simulink model "System_v2"  (R2018b)
settings: Solver=VariableStepAuto  StartTime=0.0  StopTime=stopTime  MaxStep=maxStepSize  RelTol=1e-3
InitFcn:
  | InitialisationScript_v2
values from neighbouring files (symbols this model uses):
  a_turb = -7    [InitialisationScript.m]
  AlphaEvapSteam = 3500    [InitialisationScript.m]    (also in InitialisationScript_v2.m)
  AlphaSuperSteam = 70    [InitialisationScript.m]    (also in InitialisationScript_v2.m)
  CpumpEta = 0.75    [InitialisationScript.m]    (also in InitialisationScript_v2.m)
  eta_nom = 0.8    [InitialisationScript.m]
  evapFraction = 0.95    [InitialisationScript.m]    (also in InitialisationScript_v2.m = 0.938024869451)
  fuel_mass = 10000    [InitialisationScript.m]    (also in InitialisationScript_v2.m)
  h_max = 1000    [InitialisationScript_v2.m]
  k_pipe = 2e-3    (= 0.002)    [InitialisationScript_v2.m]
  N_min = 0.35    [InitialisationScript_v2.m]
  p1 = 18    [InitialisationScript.m]
  p2 = 0.6    [InitialisationScript.m]
  pipeLength = 4    [InitialisationScript.m]    (also in InitialisationScript_v2.m = 3.66)
  pressureFG = 50*9.81*1000    (= 490500)    [InitialisationScript_v2.m]
  Q_max = 52.254728179762466    (= 52.2547281798)    [InitialisationScript_v2.m]
  returnFGdelay = 3    [InitialisationScript.m]    (also in InitialisationScript_v2.m)
  rho_ethanole = 789    [InitialisationScript.m]    (also in InitialisationScript_v2.m)
  theta1_nom = 246.76    [InitialisationScript.m]
  theta_ret = 227.95    [InitialisationScript.m]    (also in InitialisationScript_v2.m)
  thetaFuelIn = 10    [InitialisationScript.m]    (also in InitialisationScript_v2.m)
  thetaO2In = 10    [InitialisationScript.m]    (also in InitialisationScript_v2.m)
undefined symbols (not defined in the file or in its folder): AinternalEvap, AinternalSuper, AwallEvap, AwallSuper, conductivity, extDiameter, K_stodola, qmd_ref, sub, thickness
libraries: simulink x1
settings Model: Creator=Danijel  LastModifiedBy=Danijel
settings DebuggingCC: UnderSpecifiedDimensionMsg=warning

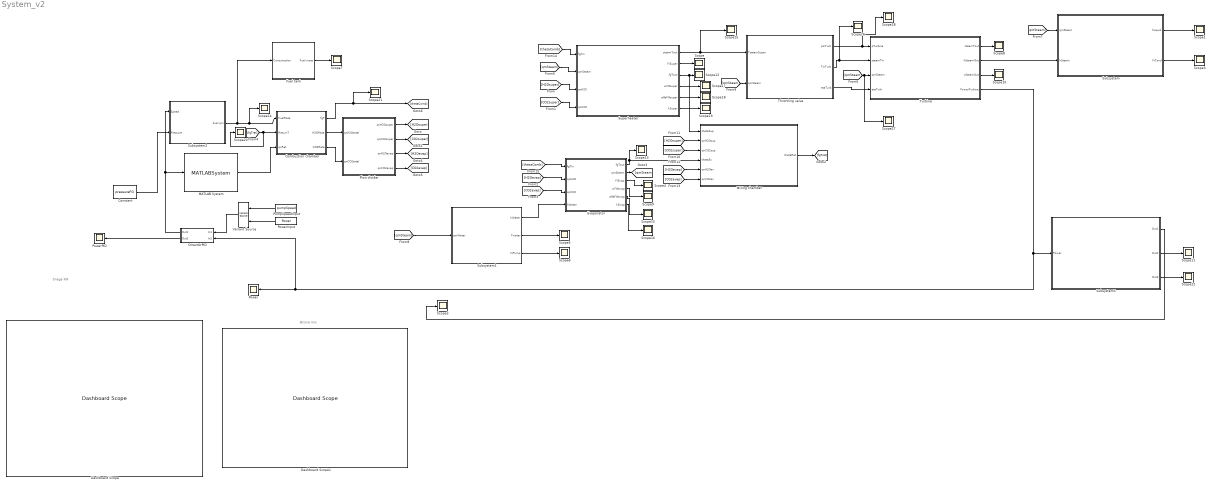
== system System_v2 ==
  note: Brzina m/s
  note: Snaga kW
  Combustion chamber : Subsystem  mask{thetaG_in=thetaFuelIn, thetaO2_in=thetaO2In, fgDelay=returnFGdelay, thetaRetInit=theta_ret}
      mask prompts: thetaG_in "Fuel temperature [°C]:"; thetaO2_in "Oxygen temperature [°C]:"; fgDelay "Flue gas return delay [s]"; thetaRetInit "Initial flue gas return temperature"
      mask help: Models fuel combustion with flue gas return
      mask TypeOptions thetaG_in: MATLAB System/thetaG_in
      mask TypeOptions thetaO2_in: MATLAB System/thetaO2_in
      mask DialogControl DescGroupVar Prompt: Combustion chamber
      mask Display: text(0.3,0.9, '{\bf\fontsize{12}Combustion}', 'texmode','on');
  Constant : Constant  Value=pressureFG
  DIrectOrPID : Subsystem  Variant=on
  Dashboard Scope : DashboardScope  Description=Turbine power  WebBlockId=277  Ymin=0  Ymax=110
  Dashboard Scope1 : DashboardScope  WebBlockId=358
  Evaporator : Subsystem  mask{p1=p1, A_evap=AwallEvap, flueGasFlowArea=AinternalEvap, pipeDiameterExternal=extDiameter, pipeThickness=thickness, AlfaS=AlphaEvapSteam, pipeConductivity=conductivity}
      mask prompts: p1 "Evaporation pressure [bar]:"; A_evap "Evaporator heat transfer area [m2]:"; flueGasFlowArea "Evaporator overall internal tube crossection area [m2]:"; pipeDiameterExternal "Evaporator pipe external diameter [m]:"; pipeThickness "Evaporator pipe thickness [m]:"; AlfaS "Evaporation heat transfer coefficient [W/m2K]:"; pipeConductivity "Tube material thermal conductivity [W/(mK)]:"
      mask help: Models steam evaporation. Calculates steam flow rate and flue gas outlet temperature.
      mask TypeOptions p1: MATLAB System2/p1
      mask TypeOptions A_evap: MATLAB System2/A_evap
      mask TypeOptions flueGasFlowArea: MATLAB System2/flueGasFlowArea
      mask TypeOptions pipeDiameterExternal: MATLAB System2/pipeDiameterExternal
      mask TypeOptions pipeThickness: MATLAB System2/pipeThickness
      mask TypeOptions AlfaS: MATLAB System2/AlfaS
      mask TypeOptions pipeConductivity: MATLAB System2/pipeConductivity
      mask DialogControl DescGroupVar Prompt: Evaporator
      mask Display: text(0.35,0.9, '{\bf\fontsize{12}Evaporator}', 'texmode','on');
  Flow divider : Subsystem  mask{evap_ratio=evapFraction}
      mask prompts: evap_ratio "Fraction of flue gases to evaporator [0-1]"
  Fuel tank : Subsystem  mask{InitialFuelMass=fuel_mass}
      mask prompts: InitialFuelMass "Initial fuel mass [kg]"
      mask Display: text(0.3,0.9, '{\bf\fontsize{12}Fuel tank}', 'texmode','on');
  MATLAB System : MATLABSystem  System=CompressorS  qmRetMin=qnRetMin  qmRetMax=qnRetMax  qmRetlow=qnRetlow  qmRethigh=qnRethigh  Nretlow=Nretlow  Nrethigh=Nrethigh  SimulateUsing=Code generation
      mask Type: CompressorS
      mask Display:
      | disp('CompressorS');
      | port_label('input',1,'N');
      | port_label('output',1,'qmRet');
  Mixing chamber : Subsystem
      mask Display: text(0.35,0.9, '{\bf\fontsize{12}Flue gas mix}', 'texmode','on');
  Power : Scope
  PowerInput : FromWorkspace  VariableName=Power  SampleTime=0
  PowerPID : Scope
  PumpSpeedInput : FromWorkspace  VariableName=pumpSpeed  SampleTime=0
  Scope{,1..22,25..28} (27 alike) : Scope
  Subsystem : Subsystem  mask{p2=p2}
      mask prompts: p2 "Condensation pressure [bar]:"
      mask help: Models steam condensation.
      mask TypeOptions p2: MATLAB System/p2
      mask DialogControl DescGroupVar Prompt: Condenser
      mask Display: text(0.4,0.9, '{\bf\fontsize{12}Condenser}', 'texmode','on');
  Subsystem1 : Subsystem  mask{p1=p1, p2=p2, eta=CpumpEta}
      mask prompts: p1 "Evaporation pressure [bar]:"; p2 "Condensation pressure [bar]:"; eta "Pump efficiency  [-]:"
      mask TypeOptions p1: MATLAB System/p1
      mask TypeOptions p2: MATLAB System/p2
      mask TypeOptions eta: MATLAB System/eta
      mask Display: text(0.27,0.92, '{\bf\fontsize{12}Condensate pump}', 'texmode','on');
  Subsystem2 : Subsystem  mask{Q_max=Q_max, h_max=h_max, n_min=N_min, rho_ethanole=rho_ethanole, k_pipe=k_pipe}
      mask prompts: Q_max "Fuel pump nominal volume flow rate [l/h]:"; h_max "Fuel pump nominal head [m]:"; n_min "Pump minimal relative speed [-]:"; rho_ethanole "Ethanole density [kg/m3]:"; k_pipe "pipe coefficient:"
      mask TypeOptions Q_max: MATLAB System/Q_max
      mask TypeOptions h_max: MATLAB System/h_max
      mask TypeOptions n_min: MATLAB System/n_min
      mask TypeOptions rho_ethanole: MATLAB System/rho_ethanole
      mask TypeOptions k_pipe: MATLAB System/k_pipe
      mask Display: text(0.3,0.9, '{\bf\fontsize{12}Fuel pump}', 'texmode','on');
  Subsystem3 : Subsystem
  Superheater : Subsystem  mask{p1=p1, A_super=AwallSuper, flueGasFlowArea=AinternalSuper, pipeDiameterExternal=extDiameter, pipeThickness=thickness, AlfaS=AlphaSuperSteam, pipeConductivity=conductivity, pipeLength=pipeLength}
      mask prompts: p1 "Evaporation pressure [bar]:"; A_super "Superheater heat transfer area [m2]:"; flueGasFlowArea "Superheater overall internal tube crossection area [m2]:"; pipeDiameterExternal "External pipe diameter [m]:"; pipeThickness "Superheater pipe thickness [m]:"; AlfaS "Superheating heat transfer coefficient [W/m2K]:"; pipeConductivity "Tube material thermal conductivity [W/(mK)]:"; pipeLength "Pipe length [m]:"
      mask help: Models steam superheating. Calculates outlet flue gas and steam temperatures.
      mask TypeOptions p1: MATLAB System3/p1
      mask TypeOptions A_super: MATLAB System3/A_super
      mask TypeOptions flueGasFlowArea: MATLAB System3/flueGasFlowArea
      mask TypeOptions pipeDiameterExternal: MATLAB System3/pipeDiameterExternal
      mask TypeOptions pipeThickness: MATLAB System3/pipeThickness
      mask TypeOptions AlfaS: MATLAB System3/AlfaS
      mask TypeOptions pipeConductivity: MATLAB System3/pipeConductivity
      mask TypeOptions pipeLength: MATLAB System3/pipeLength
      mask DialogControl DescGroupVar Prompt: Superheater
      mask Display: text(0.4,0.9, '{\bf\fontsize{12}Superheater}', 'texmode','on');
  Throttling valve : Subsystem  mask{p1=p1, p2=p2, theta1_nom=theta1_nom, qmd_nom=qmd_ref, eta_nom=eta_nom, a=a_turb, K=K_stodola}
      mask prompts: p1 "Evaporation pressure [bar]:"; p2 "Condensation pressure [bar]:"; theta1_nom "Nominal superheating temperature [°C]:"; qmd_nom "Nominal steam mass flow rate [kg/s]:"; eta_nom "Efficiency at nominal working conditions [-]:"; a "Quadratic efficiency coefficient:"; K "Stodola coefficient:"
      mask TypeOptions p1: MATLAB System/p1
      mask TypeOptions p2: MATLAB System/p2
      mask TypeOptions theta1_nom: MATLAB System/theta1_nom
      mask TypeOptions qmd_nom: MATLAB System/qmd_nom
      mask TypeOptions eta_nom: MATLAB System/eta_nom
      mask TypeOptions a: MATLAB System/a
      mask TypeOptions K: MATLAB System/K
      mask Display: text(0.35,0.9, '{\bf\fontsize{12}Throttling valve}', 'texmode','on');
  Turbine : Subsystem  mask{p_evap=p1, p2=p2}
      mask prompts: p_evap "Evaporation pressure [bar]:"; p2 "Condensation pressure [bar]:"
      mask help: Models steam expansion in tuebine. Calulates turbine power and outlet steam state.
      mask TypeOptions p_evap: MATLAB System4/p_evap
      mask TypeOptions p2: MATLAB System4/p2
      mask DialogControl DescGroupVar Prompt: Steam turbine
      mask Display: text(0.4,0.9, '{\bf\fontsize{12}Steam turbine}', 'texmode','on');
  Variant Source : VariantSource
  wires:
  [fgTret] -> Scope20/1, Combustion chamber/2(ReturnT)
  Evaporator/2(qmSteam) -> [qmSteam]
  [qmSteam] -> Superheater/2(qmSteam)
  Superheater/2(FiSuper) -> Scope/1
  [qmSteam] -> Scope27/1, Turbine/3(qmSteam)
  Turbine/1(steamTout) -> Scope8/1
  Turbine/3(xSteamOut) -> Scope10/1
  [qmSteam] -> Subsystem/1(qmSteam)
  Turbine/2(hSteamOut) -> Subsystem/2(hSteam)
  Subsystem/1(hLiquid) -> Scope1/1
  Subsystem/2(FiCond) -> Scope3/1
  Subsystem1/1(hWater) -> Evaporator/4(hWater)
  [qmSteam] -> Subsystem1/1(qmWater)
  Subsystem1/2(Twater) -> Scope5/1
  Subsystem1/3(FiPump) -> Scope6/1
  Fuel tank/1(Fuel mass) -> Scope7/1
  Superheater/1(steamTout) -> Scope25/1, Throttling valve/1(TsteamSuper)
  [qmSteam] -> Throttling valve/2(qmSteam)
  Throttling valve/1(pInTurb) -> Scope28/1, Turbine/1(pTurbine)
  Throttling valve/2(TinTurb) -> Scope26/1, Turbine/2(steamTin)
  Throttling valve/3(etaTurb) -> Turbine/4(etaTurb)
  Evaporator/1(fgTout) -> Mixing chamber/4(thetaEv), Scope13/1
  Superheater/3(fgTout) -> Mixing chamber/1(thetaSup), Scope12/1
  Combustion chamber/2(H2ORate) -> Flow divider/1(qnH2Ototal)
  Combustion chamber/3(CO2Rate) -> Flow divider/2(qnCO2total)
  Flow divider/1(qnH2Osuper) -> [H2Osuper]
  Flow divider/2(qnCO2super) -> [CO2super]
  Flow divider/3(qnH2Oevap) -> [H2Oevap]
  Flow divider/4(qnCO2evap) -> [CO2evap]
  [H2Osuper] -> Superheater/3(qnH20)
  [CO2super] -> Superheater/4(qnCO2)
  [H2Oevap] -> Evaporator/2(qnH2O)
  [CO2evap] -> Evaporator/3(qnCO2)
  [thetaComb] -> Superheater/1(fgTin)
  [thetaComb] -> Evaporator/1(fgTin)
  [H2Osuper] -> Mixing chamber/2(qnH2Osup)
  [CO2super] -> Mixing chamber/3(qnCO2sup)
  [H2Oevap] -> Mixing chamber/5(qnH2Oev)
  [CO2evap] -> Mixing chamber/6(qnCO2ev)
  Mixing chamber/1(thetaRet) -> [fgTret]
  Evaporator/3(FiEvap) -> Scope4/1
  Evaporator/4(wFGevap) -> Scope9/1
  Evaporator/5(alfaFGevap) -> Scope15/1
  Evaporator/6(kEvap) -> Scope16/1
  Superheater/4(wFGsuper) -> Scope17/1
  Superheater/5(alfaFGsuper) -> Scope18/1
  Superheater/6(kSuper) -> Scope19/1
  Combustion chamber/1(fgT) -> Scope21/1, [thetaComb]
  Turbine/4(PowerTurbine) -> Subsystem3/1("Power "), DIrectOrPID/2(In2), Power/1
  DIrectOrPID/2(Out2) -> PowerPID/1
  PowerInput/1 -> Variant Source/2
  PumpSpeedInput/1 -> Variant Source/1
  Variant Source/1 -> DIrectOrPID/1(In1)
  Subsystem2/1(Fuel qm) -> Fuel tank/1(Consumption), Scope14/1, Combustion chamber/1(FuelRate)
  DIrectOrPID/1(Out1) -> MATLAB System/1, Subsystem2/1(Speed)
  Constant/1 -> Subsystem2/2(Pressure)
  MATLAB System/1 -> Combustion chamber/3(qnRet)
  Subsystem3/1(Out1) -> Scope2/1
  Subsystem3/2(Out2) -> Scope11/1
  Subsystem3/3(Out3) -> Scope22/1

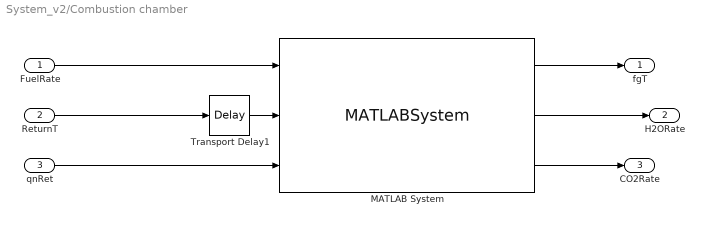
== system System_v2/Combustion chamber ==
  FuelRate : Inport
  ReturnT : Inport  Port=2
  qnRet : Inport  Port=3
  MATLAB System : MATLABSystem  System=CombustionChamberS  thetaG_in=thetaG_in  thetaO2_in=thetaO2_in  SimulateUsing=Code generation
      mask Type: CombustionChamberS
      mask Display:
      | disp('CombustionChamberS');
      | port_label('input',1,'qmG');
      | port_label('input',2,'theta_ret');
      | port_label('input',3,'qnRet');
      | port_label('output',1,'thetaFGout');
      | port_label('output',2,'qnH20out');
      | port_label('output',3,'qnCO2out');
  Transport Delay1 : TransportDelay  DelayTime=fgDelay  InitialOutput=thetaRetInit
  fgT : Outport
  H2ORate : Outport  Port=2
  CO2Rate : Outport  Port=3
  wires:
  FuelRate/1 -> MATLAB System/1
  MATLAB System/2 -> H2ORate/1
  Transport Delay1/1 -> MATLAB System/2
  MATLAB System/3 -> CO2Rate/1
  qnRet/1 -> MATLAB System/3
  MATLAB System/1 -> fgT/1
  ReturnT/1 -> Transport Delay1/1

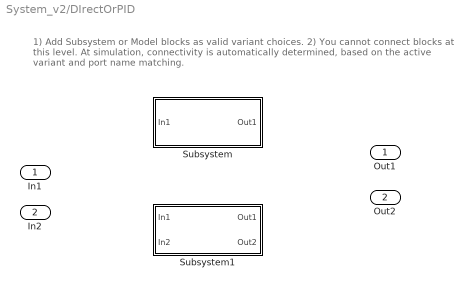
== system System_v2/DIrectOrPID ==
  note: 1) Add Subsystem or Model blocks as valid variant choices.
      | 2) You cannot connect blocks at this level. At simulation, connectivity is automatically
      | determined, based on the active variant and port name matching.
  In1 : Inport
  In2 : Inport  Port=2
  Subsystem : Subsystem  VariantControl=V==1
  Subsystem1 : Subsystem  VariantControl=V==2
  Out1 : Outport
  Out2 : Outport  Port=2

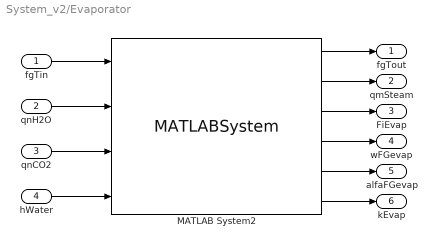
== system System_v2/Evaporator ==
  fgTin : Inport
  qnH2O : Inport  Port=2
  qnCO2 : Inport  Port=3
  hWater : Inport  Port=4
  MATLAB System2 : MATLABSystem  System=EvaporatorS  p1=p1  A_evap=A_evap  flueGasFlowArea=flueGasFlowArea  pipeDiameterExternal=pipeDiameterExternal  pipeThickness=pipeThickness  AlfaS=AlfaS  pipeConductivity=pipeConductivity  pipeLength=4  SimulateUsing=Code generation
      mask Type: EvaporatorS
      mask Display:
      | disp('EvaporatorS');
      | port_label('input',1,'theta_fg1');
      | port_label('input',2,'qnH20');
      | port_label('input',3,'qnCO2');
      | port_label('input',4,'hWater');
      | port_label('output',1,'thetaFGout');
      | port_label('output',2,'qm_d');
      | port_label('output',3,'Fi_evap');
      | port_label('output',4,'w_fg_evap');
      | port_label('output',5,'alfaFGevap');
      | port_label('output',6,'kEvap');
  fgTout : Outport
  qmSteam : Outport  Port=2
  FiEvap : Outport  Port=3
  wFGevap : Outport  Port=4
  alfaFGevap : Outport  Port=5
  kEvap : Outport  Port=6
  wires:
  MATLAB System2/1 -> fgTout/1
  fgTin/1 -> MATLAB System2/1
  MATLAB System2/3 -> FiEvap/1
  qnCO2/1 -> MATLAB System2/3
  MATLAB System2/2 -> qmSteam/1
  qnH2O/1 -> MATLAB System2/2
  hWater/1 -> MATLAB System2/4
  MATLAB System2/4 -> wFGevap/1
  MATLAB System2/5 -> alfaFGevap/1
  MATLAB System2/6 -> kEvap/1

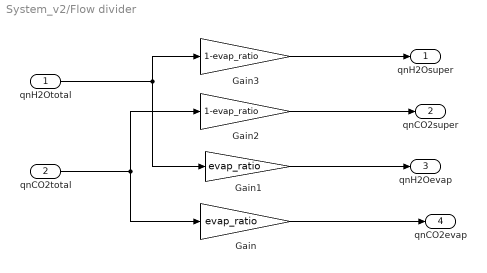
== system System_v2/Flow divider ==
  qnH2Ototal : Inport
  qnCO2total : Inport  Port=2
  Gain : Gain  Gain=evap_ratio
  Gain1 : Gain  Gain=evap_ratio
  Gain2 : Gain  Gain=1-evap_ratio
  Gain3 : Gain  Gain=1-evap_ratio
  qnH2Osuper : Outport
  qnCO2super : Outport  Port=2
  qnH2Oevap : Outport  Port=3
  qnCO2evap : Outport  Port=4
  wires:
  Gain3/1 -> qnH2Osuper/1
  Gain2/1 -> qnCO2super/1
  Gain1/1 -> qnH2Oevap/1
  qnCO2total/1 -> Gain2/1, Gain/1
  qnH2Ototal/1 -> Gain3/1, Gain1/1
  Gain/1 -> qnCO2evap/1

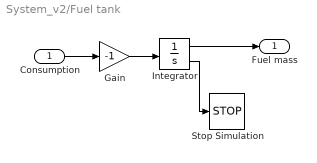
== system System_v2/Fuel tank ==
  Consumption : Inport
  Gain : Gain  Gain=-1
  Integrator : Integrator  InitialCondition=InitialFuelMass  LimitOutput=on  LowerSaturationLimit=0  ShowSaturationPort=on
  Stop Simulation : Stop
  Fuel mass : Outport
  wires:
  Integrator/2 -> Stop Simulation/1
  Gain/1 -> Integrator/1
  Integrator/1 -> Fuel mass/1
  Consumption/1 -> Gain/1

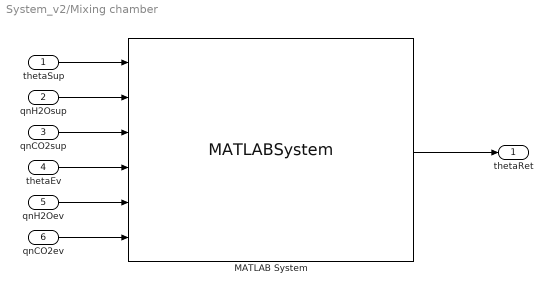
== system System_v2/Mixing chamber ==
  thetaSup : Inport
  qnH2Osup : Inport  Port=2
  qnCO2sup : Inport  Port=3
  thetaEv : Inport  Port=4
  qnH2Oev : Inport  Port=5
  qnCO2ev : Inport  Port=6
  MATLAB System : MATLABSystem  System=FlueGasMixS  SimulateUsing=Code generation
      mask Type: FlueGasMixS
      mask Display:
      | disp('FlueGasMixS');
      | port_label('input',1,'thetaSup');
      | port_label('input',2,'qnH2Osup');
      | port_label('input',3,'qnCO2sup');
      | port_label('input',4,'thetaEv');
      | port_label('input',5,'qnH2Oev');
      | port_label('input',6,'qnCO2ev');
      | port_label('output',1,'theta_ret');
  thetaRet : Outport
  wires:
  qnH2Oev/1 -> MATLAB System/5
  qnCO2ev/1 -> MATLAB System/6
  thetaSup/1 -> MATLAB System/1
  qnH2Osup/1 -> MATLAB System/2
  thetaEv/1 -> MATLAB System/4
  MATLAB System/1 -> thetaRet/1
  qnCO2sup/1 -> MATLAB System/3

== system System_v2/Subsystem ==
  qmSteam : Inport
  hSteam : Inport  Port=2
  MATLAB System : MATLABSystem  System=CondenserS  p2=p2  SimulateUsing=Code generation
      mask Type: CondenserS
      mask Display:
      | disp('CondenserS');
      | port_label('input',1,'qmSteam');
      | port_label('input',2,'hSteam');
      | port_label('output',1,'hLiquid');
      | port_label('output',2,'Fi_kond');
  hLiquid : Outport
  FiCond : Outport  Port=2
  wires:
  hSteam/1 -> MATLAB System/2
  MATLAB System/1 -> hLiquid/1
  MATLAB System/2 -> FiCond/1
  qmSteam/1 -> MATLAB System/1

== system System_v2/Subsystem1 ==
  qmWater : Inport
  MATLAB System : MATLABSystem  System=CondensatePumpS  p1=p1  p2=p2  eta=eta  SimulateUsing=Code generation
      mask Type: CondensatePumpS
      mask Display:
      | disp('CondensatePumpS');
      | port_label('input',1,'qm');
      | port_label('output',1,'hWater');
      | port_label('output',2,'waterT');
      | port_label('output',3,'FiPump');
  hWater : Outport
  Twater : Outport  Port=2
  FiPump : Outport  Port=3
  wires:
  MATLAB System/3 -> FiPump/1
  qmWater/1 -> MATLAB System/1
  MATLAB System/2 -> Twater/1
  MATLAB System/1 -> hWater/1

== system System_v2/Subsystem2 ==
  Speed : Inport
  Pressure : Inport  Port=2
  MATLAB System : MATLABSystem  System=FuelPumpPosS  Q_max=Q_max  h_max=h_max  n_min=n_min  rho_ethanole=rho_ethanole  k_pipe=k_pipe  SimulateUsing=Code generation
      mask Type: FuelPumpPosS
      mask Display:
      | disp('FuelPumpPosS');
      | port_label('input',1,'relative_speed');
      | port_label('input',2,'pressure');
      | port_label('output',1,'qm_eth');
  Fuel qm : Outport
  wires:
  Pressure/1 -> MATLAB System/2
  Speed/1 -> MATLAB System/1
  MATLAB System/1 -> Fuel qm/1

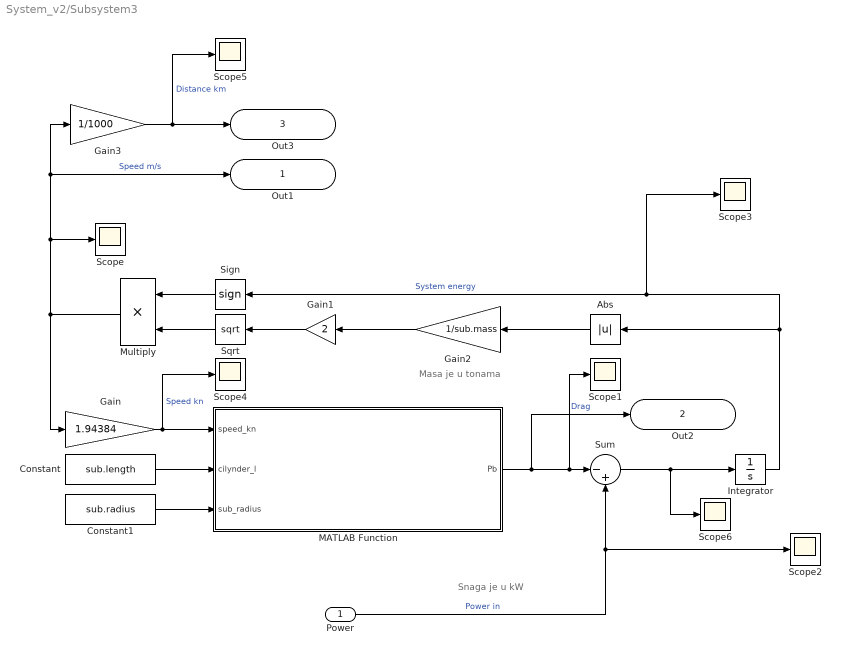
== system System_v2/Subsystem3 ==
  note: Snaga je u kW
  note: Masa je u tonama
  "Power " : Inport
  Abs : Abs
  Constant : Constant  Value=sub.length
  Constant1 : Constant  Value=sub.radius
  Gain : Gain  Gain=1.94384
  Gain1 : Gain  Gain=2
  Gain2 : Gain  Gain=1/sub.mass
  Gain3 : Gain  Gain=1/1000
  Integrator : Integrator
  MATLAB Function : MATLAB Function  TreatAsAtomicUnit=on
  Multiply : Product
  Scope{,1..6} (7 alike) : Scope
  Sign : Signum
  Sqrt : Sqrt  SaturateOnIntegerOverflow=on
  Sum : Sum  Inputs=|-+
  Out1 : Outport
  Out2 : Outport  Port=2
  Out3 : Outport  Port=3
  wires:
  Multiply/1 -> Gain/1, Out1/1, Gain3/1, Scope/1  "Speed m/s"
  "Power "/1 -> Sum/2, Scope2/1  "Power in"
  Gain1/1 -> Sqrt/1
  Constant/1 -> MATLAB Function/2(cilynder_l)
  Gain2/1 -> Gain1/1
  MATLAB Function/1(Pb) -> Out2/1, Sum/1, Scope1/1  "Drag"
  Abs/1 -> Gain2/1
  Gain/1 -> Scope4/1, MATLAB Function/1(speed_kn)  "Speed kn"
  Integrator/1 -> Scope3/1, Sign/1, Abs/1  "System energy"
  Sum/1 -> Scope6/1, Integrator/1
  Gain3/1 -> Out3/1, Scope5/1  "Distance km"
  Sign/1 -> Multiply/1
  Constant1/1 -> MATLAB Function/3(sub_radius)
  Sqrt/1 -> Multiply/2

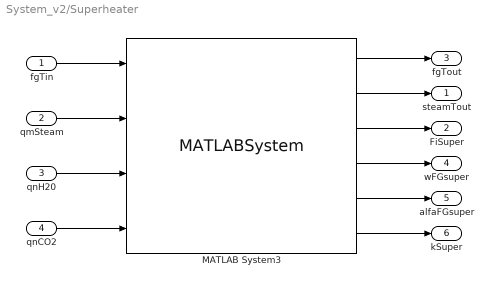
== system System_v2/Superheater ==
  fgTin : Inport
  qmSteam : Inport  Port=2
  qnH20 : Inport  Port=3
  qnCO2 : Inport  Port=4
  MATLAB System3 : MATLABSystem  System=SuperheaterS  p1=p1  A_super=A_super  flueGasFlowArea=flueGasFlowArea  pipeDiameterExternal=pipeDiameterExternal  pipeThickness=pipeThickness  AlfaS=AlfaS  pipeConductivity=pipeConductivity  pipeLength=pipeLength  SimulateUsing=Code generation
      mask Type: SuperheaterS
      mask Display:
      | disp('SuperheaterS');
      | port_label('input',1,'theta_fg2');
      | port_label('input',2,'qm_d');
      | port_label('input',3,'qnH20');
      | port_label('input',4,'qnCO2');
      | port_label('output',1,'theta_fgOut');
      | port_label('output',2,'theta1Out');
      | port_label('output',3,'Fi');
      | port_label('output',4,'w_fg_super');
      | port_label('output',5,'alfaFGsuper');
      | port_label('output',6,'kSuper');
  steamTout : Outport
  FiSuper : Outport  Port=2
  fgTout : Outport  Port=3
  wFGsuper : Outport  Port=4
  alfaFGsuper : Outport  Port=5
  kSuper : Outport  Port=6
  wires:
  fgTin/1 -> MATLAB System3/1
  MATLAB System3/3 -> FiSuper/1
  MATLAB System3/1 -> fgTout/1
  qnH20/1 -> MATLAB System3/3
  qnCO2/1 -> MATLAB System3/4
  MATLAB System3/2 -> steamTout/1
  qmSteam/1 -> MATLAB System3/2
  MATLAB System3/4 -> wFGsuper/1
  MATLAB System3/5 -> alfaFGsuper/1
  MATLAB System3/6 -> kSuper/1

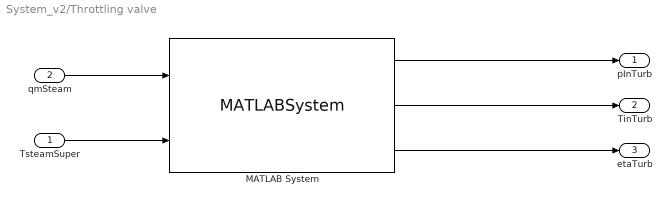
== system System_v2/Throttling valve ==
  TsteamSuper : Inport
  qmSteam : Inport  Port=2
  MATLAB System : MATLABSystem  System=ValveS  p1=p1  p2=p2  theta1_nom=theta1_nom  qmd_nom=qmd_nom  eta_nom=eta_nom  a=a  K=K  SimulateUsing=Code generation
      mask Type: ValveS
      mask Display:
      | disp('ValveS');
      | port_label('input',1,'qm_d');
      | port_label('input',2,'theta1');
      | port_label('output',1,'p_turb');
      | port_label('output',2,'theta_turb');
      | port_label('output',3,'eta_turb');
  pInTurb : Outport
  TinTurb : Outport  Port=2
  etaTurb : Outport  Port=3
  wires:
  qmSteam/1 -> MATLAB System/1
  MATLAB System/2 -> TinTurb/1
  TsteamSuper/1 -> MATLAB System/2
  MATLAB System/1 -> pInTurb/1
  MATLAB System/3 -> etaTurb/1

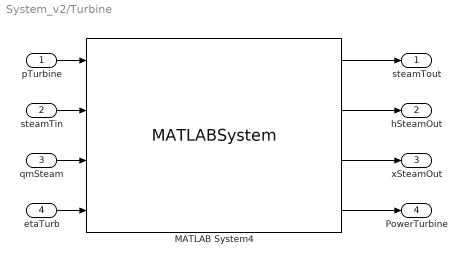
== system System_v2/Turbine ==
  pTurbine : Inport
  steamTin : Inport  Port=2
  qmSteam : Inport  Port=3
  etaTurb : Inport  Port=4
  MATLAB System4 : MATLABSystem  System=TurbineS  p_evap=p_evap  p2=p2  SimulateUsing=Code generation
      mask Type: TurbineS
      mask Display:
      | disp('TurbineS');
      | port_label('input',1,'p_turb');
      | port_label('input',2,'theta_d1');
      | port_label('input',3,'qm_d');
      | port_label('input',4,'eta_turb');
      | port_label('output',1,'thetaOut');
      | port_label('output',2,'hOut');
      | port_label('output',3,'xOut');
      | port_label('output',4,'Power');
  steamTout : Outport
  hSteamOut : Outport  Port=2
  xSteamOut : Outport  Port=3
  PowerTurbine : Outport  Port=4
  wires:
  MATLAB System4/1 -> steamTout/1
  MATLAB System4/3 -> xSteamOut/1
  MATLAB System4/2 -> hSteamOut/1
  MATLAB System4/4 -> PowerTurbine/1
  etaTurb/1 -> MATLAB System4/4
  qmSteam/1 -> MATLAB System4/3
  steamTin/1 -> MATLAB System4/2
  pTurbine/1 -> MATLAB System4/1

== system System_v2/DIrectOrPID/Subsystem ==
  In1 : Inport
  Out1 : Outport
  wires:
  In1/1 -> Out1/1

== system System_v2/DIrectOrPID/Subsystem1 ==
  In1 : Inport
  In2 : Inport  Port=2
  Regulator : Subsystem  mask{P=0.3, I=0.3, delay=1, InitialP=40, ErrorGain=1/110}
      mask prompts: P "Proportional (P):"; I "Integral (I):"; delay "Signal delay:"; InitialP "Initial power signal:"
  Out1 : Outport
  Out2 : Outport  Port=2
  wires:
  Regulator/1(Out1) -> Out1/1
  Regulator/2(Out2) -> Out2/1
  In1/1 -> Regulator/1(In1)
  In2/1 -> Regulator/2(In2)

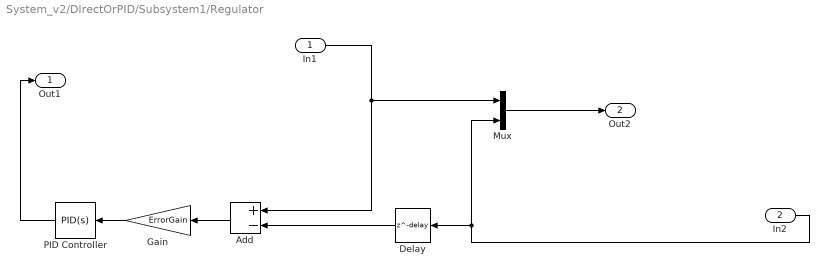
== system System_v2/DIrectOrPID/Subsystem1/Regulator ==
  In1 : Inport
  In2 : Inport  Port=2
  Add : Sum  Inputs=+-
  Delay : Delay  DelayLength=delay  InitialCondition=InitialP
  Gain : Gain  Gain=ErrorGain
  Mux : Mux  Inputs=2
  PID Controller : simulink/Continuous/PID Controller  Controller=PID  Form=Parallel  TimeDomain=Continuous-time  SampleTime=-1  IntegratorMethod=Forward Euler  FilterMethod=Forward Euler  ControllerParametersSource=internal  P=P  I=I  D=0  UseFilter=on  N=100  TunerSelectOption=Transfer Function Based (PID Tuner App)  InitialConditionSource=internal  InitialConditionForIntegrator=0  InitialConditionForFilter=0  DifferentiatorICPrevScaledInput=0  ExternalReset=none  TrackingMode=off  Kt=1  LimitOutput=on  UpperSaturationLimit=1  LowerSaturationLimit=0.36  LinearizeAsGain=off  AntiWindupMode=none  Kb=1  POutMin=[]  POutMax=[]  IOutMin=[]  IOutMax=[]  DOutMin=[]  DOutMax=[]  NOutMin=[]  NOutMax=[]  SumOutMin=[]  SumOutMax=[]  SaturationOutMin=[]  SaturationOutMax=[]  PParamMin=[]  PParamMax=[]  IParamMin=[]  IParamMax=[]  DParamMin=[]  DParamMax=[]  NParamMin=[]  NParamMax=[]  KbParamMin=[]  KbParamMax=[]  KtParamMin=[]  KtParamMax=[]  KbOutMin=[]  KbOutMax=[]  KtOutMin=[]  KtOutMax=[]  IntegratorOutMin=[]  IntegratorOutMax=[]  FilterOutMin=[]  FilterOutMax=[]  SumI1OutMin=[]  SumI1OutMax=[]  SumI2OutMin=[]  SumI2OutMax=[]  SumI3OutMin=[]  SumI3OutMax=[]  SumI4OutMin=[]  SumI4OutMax=[]  SumDOutMin=[]  SumDOutMax=[]  DifferentiatorOutMin=[]  DifferentiatorOutMax=[]  FilterDiffOutCoefMin=[]  FilterDiffOutCoefMax=[]  ReciprocalOutMin=[]  ReciprocalOutMax=[]  SumDenOutMin=[]  SumDenOutMax=[]  SumNumOutMin=[]  SumNumOutMax=[]  DivideOutMin=[]  DivideOutMax=[]  IntegratorContinuousStateAttributes=''  IntegratorStateMustResolveToSignalObject=off  IntegratorRTWStateStorageClass=Auto  FilterContinuousStateAttributes=''  FilterStateMustResolveToSignalObject=off  FilterRTWStateStorageClass=Auto  ParallelPVariant=InternalParameters  IdealPVariant=Disabled  IVariant=InternalParameters  DVariant=InternalParameters  IntegratorVariant=Continuous  SatVariant=Enabled  AWVariant=Passthrough  PCopyVariant=Disabled  TRVariant=Disabled  FdbkBlocksVariant=Forward  IdealPFdbkVariant=Disabled  SatFdbkVariant=Disabled  DerivativeFilterVariant=ContFilter  NVariant=InternalParameters  NCopyVariant=Disabled  FilterICVariant=InternalICsFilter  IntegratorICVariant=InternalICs  ExternalResetVariant=Disabled  TRSumVariant=Passthrough  SumFdbkVariant=Disabled  SumVariant=Sum_PID
  Out1 : Outport
  Out2 : Outport  Port=2
  wires:
  Gain/1 -> PID Controller/1
  Delay/1 -> Add/2
  In2/1 -> Mux/2, Delay/1
  Add/1 -> Gain/1
  In1/1 -> Add/1, Mux/1
  PID Controller/1 -> Out1/1
  Mux/1 -> Out2/1

== matlab function System_v2/Subsystem3/MATLAB Function ==
  data: speed_kn input; Pb output; cilynder_l input; sub_radius input
function Pb  = sub_power(speed_kn,cilynder_l, sub_radius)
%sub_power Summary of this function goes here
%   Detailed explanation goes here



% Densities
row = 1025; % kg/m^3 - Salt water
roc = 7850; % kg/m^3 - Steel
rop = 1300; % kg/m^3 - Plastics

% Physical constants
g = 9.81; % m/s^2

negative = 1;

if speed_kn < 0
    negative = -1;
    speed_kn = speed_kn * -1;
end

% Surface

sub_length = cilynder_l + 2 * sub_radius;

sur_cylinder = 2 * sub_radius * pi * cilynder_l;
sur_sphere =  4 * sub_radius^2 * pi;

sub_surface = sur_cylinder + sur_sphere;

% Volume

vol_cylinder = sub_radius^2 * cilynder_l * pi; % m^3
vol_sphere = 4/3 * sub_radius^3 * pi; % m^3
sub_volume = vol_cylinder + vol_sphere; % m^3

istisnina = row * sub_volume; % t

CB =  sub_volume / (sub_length * 2 * sub_radius * 2 * sub_radius); % Block coefficient





speed_ms = speed_kn * 0.514444;

ni = 0.000001187; % m^2/s - Kinematic vicscosity 
Rn = speed_ms * sub_length / ni; % Reynolds_number

CF = 0.075/(log10(Rn)-2)^2; % Friction coefficient

Fn = speed_ms /sqrt(9.08665 * sub_length);


k=-0.095+25.6 *CB/((sub_length/(2*sub_radius))^2);

CT = CF * (1 + k);

Re = CT * 0.5 * row * speed_ms^2 * sub_surface / 1000; % kW
Pe = Re * speed_ms; % kW
Pb1 = Pe/(0.5*0.98);
Pb = Pb1/0.85; % kW


Pb = Pb * negative;

end
